simulink model "MHILSimHWImpl"  (R2024a)
settings: Solver=FixedStepDiscrete  StartTime=0.0  StopTime=2e-4  FixedStep=4e-9  RelTol=1e-3
values from neighbouring files (symbols this model uses):
  cfg = tddbl_model    [HILSimModel.m]
undefined symbols (not defined in the file or in its folder): AXI4, dt, hw, ip, Lite, xc7z020clg400
libraries: hdlBasic x1497, hdlUtilities x3, vmcUtilities x1
(part 4 of 11)

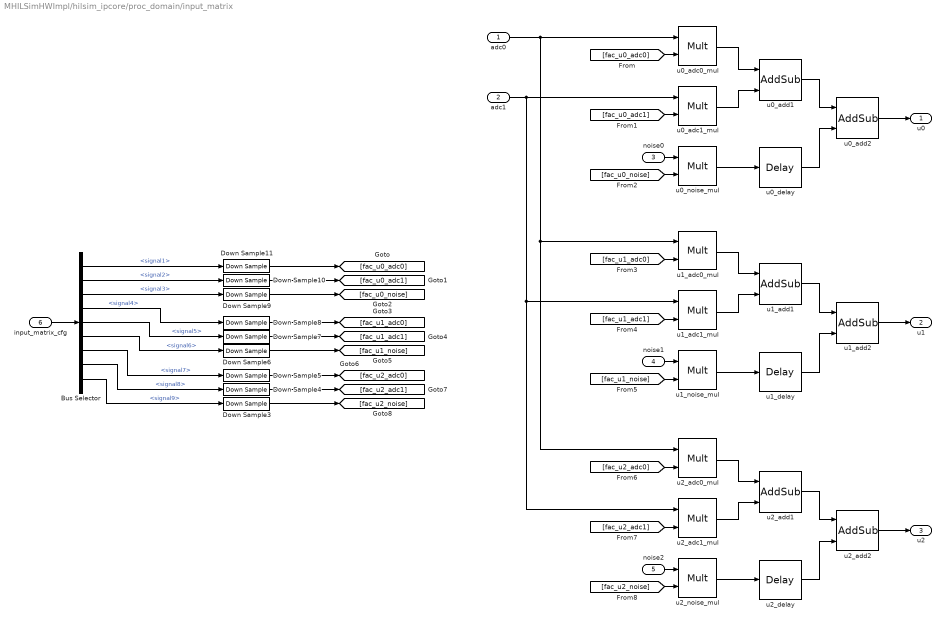
== system MHILSimHWImpl/hilsim_ipcore/proc_domain/input_matrix ==
  adc0 : Inport
  adc1 : Inport  Port=2
  noise0 : Inport  Port=3
  noise1 : Inport  Port=4
  noise2 : Inport  Port=5
  input_matrix_cfg : Inport  Port=6
  Bus Selector : BusSelector  OutputSignals=signal1,signal2,signal3,signal4,signal5,signal6,signal7,signal8,signal9
  Down Sample{3..11} (9 alike) : hdlBasic/Down Sample  sample_ratio=hw.oversample  sample_phase="Last Value of Frame  (most efficient)"  en=off  rst=off  latency=1  XmcBlockStatus=1  maskContainerNames=group1  block_type=dsamp  block_config=sysgen:Downsample_config
  u0_adc0_mul : hdlBasic/Mult  precision=User Defined  arith_type="Signed  (2's comp)"  n_bits=dt.slice.sz  bin_pt=dt.slice.bin  quantization=Truncate  overflow=Wrap  en=off  latency=3  opt_float=off  fp_mult_usage=No Usage  use_behavioral_HDL=off  opt=Speed  use_embedded=on  optimum_pipeline=off  pipeline=on  use_rpm=on  placement_style=Triangular  XmcBlockStatus=1  maskContainerNames=group1  block_type=mult  block_config=sysgen:Mult_config  block_width=598  block_height=876
  u0_adc1_mul : hdlBasic/Mult  precision=User Defined  arith_type="Signed  (2's comp)"  n_bits=dt.slice.sz  bin_pt=dt.slice.bin  quantization=Truncate  overflow=Wrap  en=off  latency=3  opt_float=off  fp_mult_usage=No Usage  use_behavioral_HDL=off  opt=Speed  use_embedded=on  optimum_pipeline=off  pipeline=on  use_rpm=on  placement_style=Triangular  XmcBlockStatus=1  maskContainerNames=group1  block_type=mult  block_config=sysgen:Mult_config  block_width=598  block_height=876
  u0_add1 : hdlBasic/AddSub  mode=Addition  use_carryin=off  use_carryout=off  en=off  latency=1  precision=User Defined  arith_type="Signed  (2's comp)"  n_bits=dt.slice.sz  bin_pt=dt.slice.bin  quantization=Truncate  overflow=Wrap  use_behavioral_HDL=off  hw_selection=Fabric  pipelined=off  XmcBlockStatus=1  maskContainerNames=tabcontainer1  block_type=addsub  block_config=sysgen:Addsub_config
  u0_add2 : hdlBasic/AddSub  mode=Addition  use_carryin=off  use_carryout=off  en=off  latency=1  precision=User Defined  arith_type="Signed  (2's comp)"  n_bits=dt.slice.sz  bin_pt=dt.slice.bin  quantization=Truncate  overflow=Wrap  use_behavioral_HDL=off  hw_selection=Fabric  pipelined=off  XmcBlockStatus=1  maskContainerNames=tabcontainer1  block_type=addsub  block_config=sysgen:Addsub_config
  u0_delay : hdlBasic/Delay  rst=off  en=off  latency=1  reg_retiming=off  XmcBlockStatus=1  maskContainerNames=group1  block_type=delay  block_config=sysgen:Delay_config
  u0_noise_mul : hdlBasic/Mult  precision=User Defined  arith_type="Signed  (2's comp)"  n_bits=dt.slice.sz  bin_pt=dt.slice.bin  quantization=Truncate  overflow=Wrap  en=off  latency=3  opt_float=off  fp_mult_usage=No Usage  use_behavioral_HDL=off  opt=Speed  use_embedded=on  optimum_pipeline=off  pipeline=on  use_rpm=on  placement_style=Triangular  XmcBlockStatus=1  maskContainerNames=group1  block_type=mult  block_config=sysgen:Mult_config  block_width=598  block_height=876
  u1_adc0_mul : hdlBasic/Mult  precision=User Defined  arith_type="Signed  (2's comp)"  n_bits=dt.slice.sz  bin_pt=dt.slice.bin  quantization=Truncate  overflow=Wrap  en=off  latency=3  opt_float=off  fp_mult_usage=No Usage  use_behavioral_HDL=off  opt=Speed  use_embedded=on  optimum_pipeline=off  pipeline=on  use_rpm=on  placement_style=Triangular  XmcBlockStatus=1  maskContainerNames=group1  block_type=mult  block_config=sysgen:Mult_config  block_width=598  block_height=876
  u1_adc1_mul : hdlBasic/Mult  precision=User Defined  arith_type="Signed  (2's comp)"  n_bits=dt.slice.sz  bin_pt=dt.slice.bin  quantization=Truncate  overflow=Wrap  en=off  latency=3  opt_float=off  fp_mult_usage=No Usage  use_behavioral_HDL=off  opt=Speed  use_embedded=on  optimum_pipeline=off  pipeline=on  use_rpm=on  placement_style=Triangular  XmcBlockStatus=1  maskContainerNames=group1  block_type=mult  block_config=sysgen:Mult_config  block_width=598  block_height=876
  u1_add1 : hdlBasic/AddSub  mode=Addition  use_carryin=off  use_carryout=off  en=off  latency=1  precision=User Defined  arith_type="Signed  (2's comp)"  n_bits=dt.slice.sz  bin_pt=dt.slice.bin  quantization=Truncate  overflow=Wrap  use_behavioral_HDL=off  hw_selection=Fabric  pipelined=off  XmcBlockStatus=1  maskContainerNames=tabcontainer1  block_type=addsub  block_config=sysgen:Addsub_config
  u1_add2 : hdlBasic/AddSub  mode=Addition  use_carryin=off  use_carryout=off  en=off  latency=1  precision=User Defined  arith_type="Signed  (2's comp)"  n_bits=dt.slice.sz  bin_pt=dt.slice.bin  quantization=Truncate  overflow=Wrap  use_behavioral_HDL=off  hw_selection=Fabric  pipelined=off  XmcBlockStatus=1  maskContainerNames=tabcontainer1  block_type=addsub  block_config=sysgen:Addsub_config
  u1_delay : hdlBasic/Delay  rst=off  en=off  latency=1  reg_retiming=off  XmcBlockStatus=1  maskContainerNames=group1  block_type=delay  block_config=sysgen:Delay_config
  u1_noise_mul : hdlBasic/Mult  precision=User Defined  arith_type="Signed  (2's comp)"  n_bits=dt.slice.sz  bin_pt=dt.slice.bin  quantization=Truncate  overflow=Wrap  en=off  latency=3  opt_float=off  fp_mult_usage=No Usage  use_behavioral_HDL=off  opt=Speed  use_embedded=on  optimum_pipeline=off  pipeline=on  use_rpm=on  placement_style=Triangular  XmcBlockStatus=1  maskContainerNames=group1  block_type=mult  block_config=sysgen:Mult_config  block_width=598  block_height=876
  u2_adc0_mul : hdlBasic/Mult  precision=User Defined  arith_type="Signed  (2's comp)"  n_bits=dt.slice.sz  bin_pt=dt.slice.bin  quantization=Truncate  overflow=Wrap  en=off  latency=3  opt_float=off  fp_mult_usage=No Usage  use_behavioral_HDL=off  opt=Speed  use_embedded=on  optimum_pipeline=off  pipeline=on  use_rpm=on  placement_style=Triangular  XmcBlockStatus=1  maskContainerNames=group1  block_type=mult  block_config=sysgen:Mult_config  block_width=598  block_height=876
  u2_adc1_mul : hdlBasic/Mult  precision=User Defined  arith_type="Signed  (2's comp)"  n_bits=dt.slice.sz  bin_pt=dt.slice.bin  quantization=Truncate  overflow=Wrap  en=off  latency=3  opt_float=off  fp_mult_usage=No Usage  use_behavioral_HDL=off  opt=Speed  use_embedded=on  optimum_pipeline=off  pipeline=on  use_rpm=on  placement_style=Triangular  XmcBlockStatus=1  maskContainerNames=group1  block_type=mult  block_config=sysgen:Mult_config  block_width=598  block_height=876
  u2_add1 : hdlBasic/AddSub  mode=Addition  use_carryin=off  use_carryout=off  en=off  latency=1  precision=User Defined  arith_type="Signed  (2's comp)"  n_bits=dt.slice.sz  bin_pt=dt.slice.bin  quantization=Truncate  overflow=Wrap  use_behavioral_HDL=off  hw_selection=Fabric  pipelined=off  XmcBlockStatus=1  maskContainerNames=tabcontainer1  block_type=addsub  block_config=sysgen:Addsub_config
  u2_add2 : hdlBasic/AddSub  mode=Addition  use_carryin=off  use_carryout=off  en=off  latency=1  precision=User Defined  arith_type="Signed  (2's comp)"  n_bits=dt.slice.sz  bin_pt=dt.slice.bin  quantization=Truncate  overflow=Wrap  use_behavioral_HDL=off  hw_selection=Fabric  pipelined=off  XmcBlockStatus=1  maskContainerNames=tabcontainer1  block_type=addsub  block_config=sysgen:Addsub_config
  u2_delay : hdlBasic/Delay  rst=off  en=off  latency=1  reg_retiming=off  XmcBlockStatus=1  maskContainerNames=group1  block_type=delay  block_config=sysgen:Delay_config
  u2_noise_mul : hdlBasic/Mult  precision=User Defined  arith_type="Signed  (2's comp)"  n_bits=dt.slice.sz  bin_pt=dt.slice.bin  quantization=Truncate  overflow=Wrap  en=off  latency=3  opt_float=off  fp_mult_usage=No Usage  use_behavioral_HDL=off  opt=Speed  use_embedded=on  optimum_pipeline=off  pipeline=on  use_rpm=on  placement_style=Triangular  XmcBlockStatus=1  maskContainerNames=group1  block_type=mult  block_config=sysgen:Mult_config  block_width=598  block_height=876
  u0 : Outport
  u1 : Outport  Port=2
  u2 : Outport  Port=3
  wires:
  u0_add1/1 -> u0_add2/1
  u0_adc0_mul/1 -> u0_add1/1
  u0_adc1_mul/1 -> u0_add1/2
  u0_noise_mul/1 -> u0_delay/1
  u0_add2/1 -> u0/1
  u1_add1/1 -> u1_add2/1
  u1_adc1_mul/1 -> u1_add1/2
  u1_adc0_mul/1 -> u1_add1/1
  u1_noise_mul/1 -> u1_delay/1
  u2_add1/1 -> u2_add2/1
  u2_adc1_mul/1 -> u2_add1/2
  u2_adc0_mul/1 -> u2_add1/1
  u2_noise_mul/1 -> u2_delay/1
  adc0/1 -> u0_adc0_mul/1, u2_adc0_mul/1, u1_adc0_mul/1
  adc1/1 -> u0_adc1_mul/1, u2_adc1_mul/1, u1_adc1_mul/1
  u1_add2/1 -> u1/1
  u2_add2/1 -> u2/1
  [fac_u0_adc0] -> u0_adc0_mul/2
  [fac_u0_adc1] -> u0_adc1_mul/2
  [fac_u0_noise] -> u0_noise_mul/2
  [fac_u1_adc0] -> u1_adc0_mul/2
  [fac_u1_adc1] -> u1_adc1_mul/2
  [fac_u1_noise] -> u1_noise_mul/2
  [fac_u2_adc0] -> u2_adc0_mul/2
  [fac_u2_noise] -> u2_noise_mul/2
  [fac_u2_adc1] -> u2_adc1_mul/2
  Bus Selector/1 -> Down Sample11/1  "<signal1>"
  Bus Selector/2 -> Down Sample10/1  "<signal2>"
  Bus Selector/3 -> Down Sample9/1  "<signal3>"
  Bus Selector/9 -> Down Sample3/1  "<signal9>"
  Bus Selector/8 -> Down Sample4/1  "<signal8>"
  Bus Selector/7 -> Down Sample5/1  "<signal7>"
  Bus Selector/6 -> Down Sample6/1  "<signal6>"
  Bus Selector/5 -> Down Sample7/1  "<signal5>"
  Bus Selector/4 -> Down Sample8/1  "<signal4>"
  input_matrix_cfg/1 -> Bus Selector/1
  Down Sample3/1 -> [fac_u2_noise]
  Down Sample4/1 -> [fac_u2_adc1]
  Down Sample5/1 -> [fac_u2_adc0]
  Down Sample7/1 -> [fac_u1_adc1]
  Down Sample8/1 -> [fac_u1_adc0]
  Down Sample6/1 -> [fac_u1_noise]
  Down Sample11/1 -> [fac_u0_adc0]
  Down Sample9/1 -> [fac_u0_noise]
  Down Sample10/1 -> [fac_u0_adc1]
  u0_delay/1 -> u0_add2/2
  u1_delay/1 -> u1_add2/2
  u2_delay/1 -> u2_add2/2
  noise0/1 -> u0_noise_mul/1
  noise1/1 -> u1_noise_mul/1
  noise2/1 -> u2_noise_mul/1

== system MHILSimHWImpl/hilsim_ipcore/proc_domain/input_shutoff ==
  enable : Inport
  u0_in : Inport  Port=2
  u1_in : Inport  Port=3
  u2_in : Inport  Port=4
  Constant1 : hdlBasic/Constant  const=0  gui_display_data_type=Fixed-point  arith_type=Signed (2's comp)  n_bits=dt.slice.sz  bin_pt=dt.slice.bin  preci_type=Single  exp_width=8  frac_width=24  explicit_period=off  period=1  XmcBlockStatus=1  maskContainerNames=tabcontainer1  block_type=constant  block_config=sysgen:Constant_config
  Constant2 : hdlBasic/Constant  const=0  gui_display_data_type=Fixed-point  arith_type=Signed (2's comp)  n_bits=dt.slice.sz  bin_pt=dt.slice.bin  preci_type=Single  exp_width=8  frac_width=24  explicit_period=off  period=1  XmcBlockStatus=1  maskContainerNames=tabcontainer1  block_type=constant  block_config=sysgen:Constant_config
  Constant3 : hdlBasic/Constant  const=0  gui_display_data_type=Fixed-point  arith_type=Signed (2's comp)  n_bits=dt.slice.sz  bin_pt=dt.slice.bin  preci_type=Single  exp_width=8  frac_width=24  explicit_period=off  period=1  XmcBlockStatus=1  maskContainerNames=tabcontainer1  block_type=constant  block_config=sysgen:Constant_config
  mux_u0 : hdlBasic/Mux  inputs=2  en=off  latency=0  precision=Full  arith_type=Unsigned  n_bits=16  bin_pt=14  quantization=Truncate  overflow=Wrap  XmcBlockStatus=1  maskContainerNames=tabcontainer1  block_type=mux  block_config=sysgen:Mux_config
  mux_u1 : hdlBasic/Mux  inputs=2  en=off  latency=0  precision=Full  arith_type=Unsigned  n_bits=16  bin_pt=14  quantization=Truncate  overflow=Wrap  XmcBlockStatus=1  maskContainerNames=tabcontainer1  block_type=mux  block_config=sysgen:Mux_config
  mux_u2 : hdlBasic/Mux  inputs=2  en=off  latency=0  precision=Full  arith_type=Unsigned  n_bits=16  bin_pt=14  quantization=Truncate  overflow=Wrap  XmcBlockStatus=1  maskContainerNames=tabcontainer1  block_type=mux  block_config=sysgen:Mux_config
  u0_out : Outport
  u1_out : Outport  Port=2
  u2_out : Outport  Port=3
  wires:
  Constant1/1 -> mux_u0/2
  Constant2/1 -> mux_u1/2
  Constant3/1 -> mux_u2/2
  u0_in/1 -> mux_u0/3
  enable/1 -> mux_u2/1, mux_u1/1, mux_u0/1
  u1_in/1 -> mux_u1/3
  u2_in/1 -> mux_u2/3
  mux_u0/1 -> u0_out/1
  mux_u1/1 -> u1_out/1
  mux_u2/1 -> u2_out/1

== system MHILSimHWImpl/hilsim_ipcore/proc_domain/nlf_lut_configurator ==
  note: Rising-Edge Trigger for Write-Enable
  procclk_lutcfg_addr : Inport
  procclk_lutcfg_data_in : Inport  Port=2
  procclk_lutcfg_we : Inport  Port=3
  cfg_nlf_start : Inport  Port=4
  Constant : hdlBasic/Constant  const=1.0  gui_display_data_type=Boolean  arith_type=Boolean  n_bits=16  bin_pt=14  preci_type=Single  exp_width=8  frac_width=24  explicit_period=off  period=1  XmcBlockStatus=1  maskContainerNames=tabcontainer1  block_type=constant  block_config=sysgen:Constant_config
  Constant1 : hdlBasic/Constant  const=1.0  gui_display_data_type=Fixed-point  arith_type=Unsigned  n_bits=ip.f_nlf.lut_addr_bits  bin_pt=0  preci_type=Single  exp_width=8  frac_width=24  explicit_period=off  period=1  XmcBlockStatus=1  maskContainerNames=tabcontainer1  block_type=constant  block_config=sysgen:Constant_config
  Constant2 : hdlBasic/Constant  const=ip.f_nlf.lut_sz-1  gui_display_data_type=Fixed-point  arith_type=Unsigned  n_bits=ip.f_nlf.lut_addr_bits  bin_pt=0  preci_type=Single  exp_width=8  frac_width=24  explicit_period=off  period=1  XmcBlockStatus=1  maskContainerNames=tabcontainer1  block_type=constant  block_config=sysgen:Constant_config
  Constant3 : hdlBasic/Constant  const=1.0  gui_display_data_type=Boolean  arith_type=Boolean  n_bits=16  bin_pt=14  preci_type=Single  exp_width=8  frac_width=24  explicit_period=off  period=1  XmcBlockStatus=1  maskContainerNames=tabcontainer1  block_type=constant  block_config=sysgen:Constant_config
  Delay : hdlBasic/Delay  rst=off  en=off  latency=1  reg_retiming=off  XmcBlockStatus=1  maskContainerNames=group1  block_type=delay  block_config=sysgen:Delay_config
  Delay1 : hdlBasic/Delay  rst=off  en=off  latency=1  reg_retiming=off  XmcBlockStatus=1  maskContainerNames=group1  block_type=delay  block_config=sysgen:Delay_config
  Mux : hdlBasic/Mux  inputs=2  en=off  latency=0  precision=Full  arith_type=Unsigned  n_bits=16  bin_pt=14  quantization=Truncate  overflow=Wrap  XmcBlockStatus=1  maskContainerNames=tabcontainer1  block_type=mux  block_config=sysgen:Mux_config
  Mux1 : hdlBasic/Mux  inputs=2  en=off  latency=0  precision=Full  arith_type=Unsigned  n_bits=16  bin_pt=14  quantization=Truncate  overflow=Wrap  XmcBlockStatus=1  maskContainerNames=tabcontainer1  block_type=mux  block_config=sysgen:Mux_config
  Register : hdlBasic/Register  init=0  rst=on  en=off  XmcBlockStatus=1  maskContainerNames=tabcontainer1  block_type=register  block_config=sysgen:Register_config
  Register1 : hdlBasic/Register  init=0  rst=on  en=off  XmcBlockStatus=1  maskContainerNames=tabcontainer1  block_type=register  block_config=sysgen:Register_config
  Relational : hdlBasic/Relational  mode=a=b  op_type=Bool  en=off  latency=1  XmcBlockStatus=1  maskContainerNames=tabcontainer1  block_type=relational  block_config=sysgen:Relational_config
  Terminator : Terminator
  addr_counter : hdlBasic/Accumulator  operation=Add  n_bits=ip.f_nlf.lut_addr_bits  overflow=Wrap  scale=1  rst=on  hasbypass=off  en=on  latency=1  msb_inp=100  msb=100  lsb=-100  use_behavioral_HDL=on  implementation=Fabric  XmcBlockStatus=1  maskContainerNames=group3  block_type=accum  block_config=sysgen:Accum_config  block_width=566  block_height=845
  bool_zero : hdlBasic/Constant  const=0  gui_display_data_type=Boolean  arith_type=Boolean  n_bits=16  bin_pt=14  preci_type=Single  exp_width=8  frac_width=24  explicit_period=off  period=1  XmcBlockStatus=1  maskContainerNames=tabcontainer1  block_type=constant  block_config=sysgen:Constant_config
  cfg_we_and : hdlBasic/Logical  logical_function=AND  inputs=2  en=off  latency=0  precision=Full  arith_type=Unsigned  n_bits=16  bin_pt=0  align_bp=on  overflow=[]  quantization=[]  XmcBlockStatus=1  maskContainerNames=tabcontainer1  block_type=logical  block_config=sysgen:Logical_config
  cfg_we_inv : hdlBasic/Inverter  en=off  latency=1  XmcBlockStatus=1  maskContainerNames=group2  block_type=inv  block_config=sysgen:Inverter_config
  tmp_lut : hdlBasic/Dual Port RAM  depth=ip.f_nlf.lut_sz  initVector=cfg.slice1.x_nlf.lut  distributed_mem=Block RAM  init_a=0  init_b=0  rst_a=off  rst_b=off  en_a=off  en_b=off  latency=1  write_mode_A=Read After Write  write_mode_B=Read After Write  explicit_period=[]  period=[]  simulation_type=fast_sim  XmcBlockStatus=1  maskContainerNames=tabcontainer1  block_type=dpram  block_config=sysgen:Dpram_config  optimize=Area
      settings: infoedit=[]
  zero_nlf_din : hdlBasic/Constant  const=0  gui_display_data_type=Fixed-point  arith_type=Signed (2's comp)  n_bits=dt.nlf.sz  bin_pt=dt.nlf.bin  preci_type=Single  exp_width=8  frac_width=24  explicit_period=off  period=1  XmcBlockStatus=1  maskContainerNames=tabcontainer1  block_type=constant  block_config=sysgen:Constant_config
  procclk_cfgbus_addr : Outport
  procclk_cfgbus_data : Outport  Port=2
  procclk_cfgbus_we : Outport  Port=3
  cfg_nlf_done : Outport  Port=4
  wires:
  procclk_lutcfg_data_in/1 -> tmp_lut/2
  procclk_lutcfg_addr/1 -> tmp_lut/1
  tmp_lut/1 -> Terminator/1
  tmp_lut/2 -> procclk_cfgbus_data/1
  cfg_nlf_start/1 -> Register1/2, Mux/1
  Mux/1 -> Register/1
  Register/1 -> addr_counter/3, Delay1/1, Mux/2
  Constant/1 -> Mux/3
  Constant1/1 -> addr_counter/1
  addr_counter/1 -> Delay/1, tmp_lut/4, Relational/1
  Relational/1 -> addr_counter/2, Mux1/1, Register/2  "cfg_nlf_last_addr"
  Constant2/1 -> Relational/2
  bool_zero/1 -> tmp_lut/6
  zero_nlf_din/1 -> tmp_lut/5
  cfg_we_and/1 -> tmp_lut/3
  cfg_we_inv/1 -> cfg_we_and/1
  procclk_lutcfg_we/1 -> cfg_we_and/2, cfg_we_inv/1
  Mux1/1 -> Register1/1
  Register1/1 -> cfg_nlf_done/1, Mux1/2
  Constant3/1 -> Mux1/3
  Delay/1 -> procclk_cfgbus_addr/1
  Delay1/1 -> procclk_cfgbus_we/1

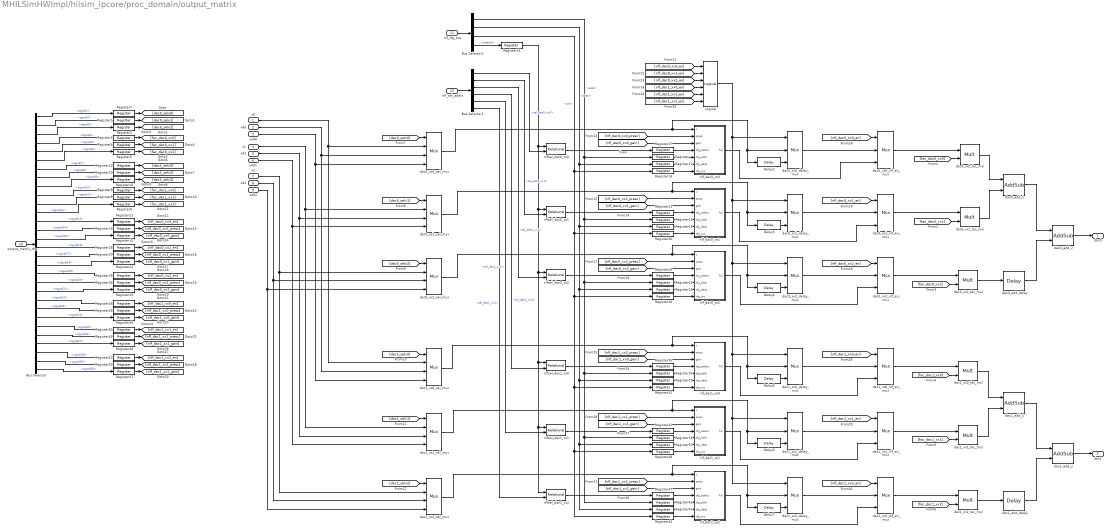
== system MHILSimHWImpl/hilsim_ipcore/proc_domain/output_matrix ==
  x0 : Inport
  xd0 : Inport  Port=2
  xdd0 : Inport  Port=3
  x1 : Inport  Port=4
  xd1 : Inport  Port=5
  xdd1 : Inport  Port=6
  x2 : Inport  Port=7
  xd2 : Inport  Port=8
  xdd2 : Inport  Port=9
  output_matrix_cfg : Inport  Port=10
  nlf_cfg_bus : Inport  Port=11
  nlf_sel_addrs : Inport  Port=12
  Bus Selector : BusSelector  OutputSignals=signal1,signal2,signal3,signal4,signal5,signal6,signal7,signal8,signal9,signal10,signal11,signal12,signal13,signal14,signal15,signal16,signal17,signal18,signal19,signal20,signal21,signal22,signal23,signal24,signal25,signal26,signal27,signal28,signal29,signal30
  Bus Selector1 : BusSelector  OutputSignals=sel_dac0_xx0,sel_dac0_xx1,sel_dac0_xx2,sel_dac1_xx0,sel_dac1_xx1,sel_dac1_xx2
  Bus Selector2 : BusSelector  OutputSignals=addr,data,we,seladdr
  Delay{2..7} (6 alike) : hdlBasic/Delay  rst=off  en=off  latency=12  reg_retiming=off  XmcBlockStatus=1  maskContainerNames=group1  block_type=delay  block_config=sysgen:Delay_config
  Logical : hdlBasic/Logical  logical_function=OR  inputs=6  en=off  latency=0  precision=Full  arith_type=Unsigned  n_bits=16  bin_pt=0  align_bp=on  overflow=[]  quantization=[]  XmcBlockStatus=1  maskContainerNames=tabcontainer1  block_type=logical  block_config=sysgen:Logical_config
  Register{,1..54} (55 alike) : hdlBasic/Register  init=0  rst=off  en=off  XmcBlockStatus=1  maskContainerNames=tabcontainer1  block_type=register  block_config=sysgen:Register_config
  dac0_add_1 : hdlBasic/AddSub  mode=Addition  use_carryin=off  use_carryout=off  en=off  latency=1  precision=User Defined  arith_type="Signed  (2's comp)"  n_bits=dt.slice.sz  bin_pt=dt.slice.bin  quantization=Truncate  overflow=Wrap  use_behavioral_HDL=off  hw_selection=Fabric  pipelined=off  XmcBlockStatus=1  maskContainerNames=tabcontainer1  block_type=addsub  block_config=sysgen:Addsub_config
  dac0_add_2 : hdlBasic/AddSub  mode=Addition  use_carryin=off  use_carryout=off  en=off  latency=1  precision=User Defined  arith_type="Signed  (2's comp)"  n_bits=dt.slice.sz  bin_pt=dt.slice.bin  quantization=Truncate  overflow=Wrap  use_behavioral_HDL=off  hw_selection=Fabric  pipelined=off  XmcBlockStatus=1  maskContainerNames=tabcontainer1  block_type=addsub  block_config=sysgen:Addsub_config
  dac0_add_delay : hdlBasic/Delay  rst=off  en=off  latency=1  reg_retiming=off  XmcBlockStatus=1  maskContainerNames=group1  block_type=delay  block_config=sysgen:Delay_config
  dac0_xx0_delay_mux : hdlBasic/Mux  inputs=2  en=off  latency=0  precision=Full  arith_type=Unsigned  n_bits=16  bin_pt=14  quantization=Truncate  overflow=Wrap  XmcBlockStatus=1  maskContainerNames=tabcontainer1  block_type=mux  block_config=sysgen:Mux_config
  dac0_xx0_fac_mul : hdlBasic/Mult  precision=User Defined  arith_type="Signed  (2's comp)"  n_bits=dt.slice.sz  bin_pt=dt.slice.bin  quantization=Truncate  overflow=Wrap  en=off  latency=3  opt_float=off  fp_mult_usage=No Usage  use_behavioral_HDL=off  opt=Speed  use_embedded=on  optimum_pipeline=off  pipeline=on  use_rpm=on  placement_style=Triangular  XmcBlockStatus=1  maskContainerNames=group1  block_type=mult  block_config=sysgen:Mult_config  block_width=598  block_height=876
  dac0_xx0_nlf_en_mux : hdlBasic/Mux  inputs=2  en=off  latency=1  precision=Full  arith_type=Unsigned  n_bits=16  bin_pt=14  quantization=Truncate  overflow=Wrap  XmcBlockStatus=1  maskContainerNames=tabcontainer1  block_type=mux  block_config=sysgen:Mux_config
  dac0_xx0_sel_mux : hdlBasic/Mux  inputs=3  en=off  latency=1  precision=Full  arith_type=Unsigned  n_bits=16  bin_pt=14  quantization=Truncate  overflow=Wrap  XmcBlockStatus=1  maskContainerNames=tabcontainer1  block_type=mux  block_config=sysgen:Mux_config
  dac0_xx1_delay_mux : hdlBasic/Mux  inputs=2  en=off  latency=0  precision=Full  arith_type=Unsigned  n_bits=16  bin_pt=14  quantization=Truncate  overflow=Wrap  XmcBlockStatus=1  maskContainerNames=tabcontainer1  block_type=mux  block_config=sysgen:Mux_config
  dac0_xx1_fac_mul : hdlBasic/Mult  precision=User Defined  arith_type="Signed  (2's comp)"  n_bits=dt.slice.sz  bin_pt=dt.slice.bin  quantization=Truncate  overflow=Wrap  en=off  latency=3  opt_float=off  fp_mult_usage=No Usage  use_behavioral_HDL=off  opt=Speed  use_embedded=on  optimum_pipeline=off  pipeline=on  use_rpm=on  placement_style=Triangular  XmcBlockStatus=1  maskContainerNames=group1  block_type=mult  block_config=sysgen:Mult_config  block_width=598  block_height=876
  dac0_xx1_nlf_en_mux : hdlBasic/Mux  inputs=2  en=off  latency=1  precision=Full  arith_type=Unsigned  n_bits=16  bin_pt=14  quantization=Truncate  overflow=Wrap  XmcBlockStatus=1  maskContainerNames=tabcontainer1  block_type=mux  block_config=sysgen:Mux_config
  dac0_xx1_sel_mux : hdlBasic/Mux  inputs=3  en=off  latency=1  precision=Full  arith_type=Unsigned  n_bits=16  bin_pt=14  quantization=Truncate  overflow=Wrap  XmcBlockStatus=1  maskContainerNames=tabcontainer1  block_type=mux  block_config=sysgen:Mux_config
  dac0_xx2_delay_mux : hdlBasic/Mux  inputs=2  en=off  latency=0  precision=Full  arith_type=Unsigned  n_bits=16  bin_pt=14  quantization=Truncate  overflow=Wrap  XmcBlockStatus=1  maskContainerNames=tabcontainer1  block_type=mux  block_config=sysgen:Mux_config
  dac0_xx2_fac_mul : hdlBasic/Mult  precision=User Defined  arith_type="Signed  (2's comp)"  n_bits=dt.slice.sz  bin_pt=dt.slice.bin  quantization=Truncate  overflow=Wrap  en=off  latency=3  opt_float=off  fp_mult_usage=No Usage  use_behavioral_HDL=off  opt=Speed  use_embedded=on  optimum_pipeline=off  pipeline=on  use_rpm=on  placement_style=Triangular  XmcBlockStatus=1  maskContainerNames=group1  block_type=mult  block_config=sysgen:Mult_config  block_width=598  block_height=876
  dac0_xx2_nlf_en_mux : hdlBasic/Mux  inputs=2  en=off  latency=1  precision=Full  arith_type=Unsigned  n_bits=16  bin_pt=14  quantization=Truncate  overflow=Wrap  XmcBlockStatus=1  maskContainerNames=tabcontainer1  block_type=mux  block_config=sysgen:Mux_config
  dac0_xx2_sel_mux : hdlBasic/Mux  inputs=3  en=off  latency=1  precision=Full  arith_type=Unsigned  n_bits=16  bin_pt=14  quantization=Truncate  overflow=Wrap  XmcBlockStatus=1  maskContainerNames=tabcontainer1  block_type=mux  block_config=sysgen:Mux_config
  dac1_add_1 : hdlBasic/AddSub  mode=Addition  use_carryin=off  use_carryout=off  en=off  latency=1  precision=User Defined  arith_type="Signed  (2's comp)"  n_bits=dt.slice.sz  bin_pt=dt.slice.bin  quantization=Truncate  overflow=Wrap  use_behavioral_HDL=off  hw_selection=Fabric  pipelined=off  XmcBlockStatus=1  maskContainerNames=tabcontainer1  block_type=addsub  block_config=sysgen:Addsub_config
  dac1_add_2 : hdlBasic/AddSub  mode=Addition  use_carryin=off  use_carryout=off  en=off  latency=1  precision=User Defined  arith_type="Signed  (2's comp)"  n_bits=dt.slice.sz  bin_pt=dt.slice.bin  quantization=Truncate  overflow=Wrap  use_behavioral_HDL=off  hw_selection=Fabric  pipelined=off  XmcBlockStatus=1  maskContainerNames=tabcontainer1  block_type=addsub  block_config=sysgen:Addsub_config
  dac1_add_delay : hdlBasic/Delay  rst=off  en=off  latency=1  reg_retiming=off  XmcBlockStatus=1  maskContainerNames=group1  block_type=delay  block_config=sysgen:Delay_config
  dac1_xx0_delay_mux : hdlBasic/Mux  inputs=2  en=off  latency=0  precision=Full  arith_type=Unsigned  n_bits=16  bin_pt=14  quantization=Truncate  overflow=Wrap  XmcBlockStatus=1  maskContainerNames=tabcontainer1  block_type=mux  block_config=sysgen:Mux_config
  dac1_xx0_fac_mul : hdlBasic/Mult  precision=User Defined  arith_type="Signed  (2's comp)"  n_bits=dt.slice.sz  bin_pt=dt.slice.bin  quantization=Truncate  overflow=Wrap  en=off  latency=3  opt_float=off  fp_mult_usage=No Usage  use_behavioral_HDL=off  opt=Speed  use_embedded=on  optimum_pipeline=off  pipeline=on  use_rpm=on  placement_style=Triangular  XmcBlockStatus=1  maskContainerNames=group1  block_type=mult  block_config=sysgen:Mult_config  block_width=598  block_height=876
  dac1_xx0_nlf_en_mux : hdlBasic/Mux  inputs=2  en=off  latency=1  precision=Full  arith_type=Unsigned  n_bits=16  bin_pt=14  quantization=Truncate  overflow=Wrap  XmcBlockStatus=1  maskContainerNames=tabcontainer1  block_type=mux  block_config=sysgen:Mux_config
  dac1_xx0_sel_mux : hdlBasic/Mux  inputs=3  en=off  latency=1  precision=Full  arith_type=Unsigned  n_bits=16  bin_pt=14  quantization=Truncate  overflow=Wrap  XmcBlockStatus=1  maskContainerNames=tabcontainer1  block_type=mux  block_config=sysgen:Mux_config
  dac1_xx1_delay_mux : hdlBasic/Mux  inputs=2  en=off  latency=0  precision=Full  arith_type=Unsigned  n_bits=16  bin_pt=14  quantization=Truncate  overflow=Wrap  XmcBlockStatus=1  maskContainerNames=tabcontainer1  block_type=mux  block_config=sysgen:Mux_config
  dac1_xx1_fac_mul : hdlBasic/Mult  precision=User Defined  arith_type="Signed  (2's comp)"  n_bits=dt.slice.sz  bin_pt=dt.slice.bin  quantization=Truncate  overflow=Wrap  en=off  latency=3  opt_float=off  fp_mult_usage=No Usage  use_behavioral_HDL=off  opt=Speed  use_embedded=on  optimum_pipeline=off  pipeline=on  use_rpm=on  placement_style=Triangular  XmcBlockStatus=1  maskContainerNames=group1  block_type=mult  block_config=sysgen:Mult_config  block_width=598  block_height=876
  dac1_xx1_nlf_en_mux : hdlBasic/Mux  inputs=2  en=off  latency=1  precision=Full  arith_type=Unsigned  n_bits=16  bin_pt=14  quantization=Truncate  overflow=Wrap  XmcBlockStatus=1  maskContainerNames=tabcontainer1  block_type=mux  block_config=sysgen:Mux_config
  dac1_xx1_sel_mux : hdlBasic/Mux  inputs=3  en=off  latency=1  precision=Full  arith_type=Unsigned  n_bits=16  bin_pt=14  quantization=Truncate  overflow=Wrap  XmcBlockStatus=1  maskContainerNames=tabcontainer1  block_type=mux  block_config=sysgen:Mux_config
  dac1_xx2_delay_mux : hdlBasic/Mux  inputs=2  en=off  latency=0  precision=Full  arith_type=Unsigned  n_bits=16  bin_pt=14  quantization=Truncate  overflow=Wrap  XmcBlockStatus=1  maskContainerNames=tabcontainer1  block_type=mux  block_config=sysgen:Mux_config
  dac1_xx2_fac_mul : hdlBasic/Mult  precision=User Defined  arith_type="Signed  (2's comp)"  n_bits=dt.slice.sz  bin_pt=dt.slice.bin  quantization=Truncate  overflow=Wrap  en=off  latency=3  opt_float=off  fp_mult_usage=No Usage  use_behavioral_HDL=off  opt=Speed  use_embedded=on  optimum_pipeline=off  pipeline=on  use_rpm=on  placement_style=Triangular  XmcBlockStatus=1  maskContainerNames=group1  block_type=mult  block_config=sysgen:Mult_config  block_width=598  block_height=876
  dac1_xx2_nlf_en_mux : hdlBasic/Mux  inputs=2  en=off  latency=1  precision=Full  arith_type=Unsigned  n_bits=16  bin_pt=14  quantization=Truncate  overflow=Wrap  XmcBlockStatus=1  maskContainerNames=tabcontainer1  block_type=mux  block_config=sysgen:Mux_config
  dac1_xx2_sel_mux : hdlBasic/Mux  inputs=3  en=off  latency=1  precision=Full  arith_type=Unsigned  n_bits=16  bin_pt=14  quantization=Truncate  overflow=Wrap  XmcBlockStatus=1  maskContainerNames=tabcontainer1  block_type=mux  block_config=sysgen:Mux_config
  nlf_dac0_xx0 : Subsystem
  nlf_dac0_xx1 : Subsystem
  nlf_dac0_xx2 : Subsystem
  nlf_dac1_xx0 : Subsystem
  nlf_dac1_xx1 : Subsystem
  nlf_dac1_xx2 : Subsystem
  nlfsel_dac0_xx0 : hdlBasic/Relational  mode=a=b  op_type=Bool  en=off  latency=1  XmcBlockStatus=1  maskContainerNames=tabcontainer1  block_type=relational  block_config=sysgen:Relational_config
  nlfsel_dac0_xx1 : hdlBasic/Relational  mode=a=b  op_type=Bool  en=off  latency=1  XmcBlockStatus=1  maskContainerNames=tabcontainer1  block_type=relational  block_config=sysgen:Relational_config
  nlfsel_dac0_xx2 : hdlBasic/Relational  mode=a=b  op_type=Bool  en=off  latency=1  XmcBlockStatus=1  maskContainerNames=tabcontainer1  block_type=relational  block_config=sysgen:Relational_config
  nlfsel_dac1_xx0 : hdlBasic/Relational  mode=a=b  op_type=Bool  en=off  latency=1  XmcBlockStatus=1  maskContainerNames=tabcontainer1  block_type=relational  block_config=sysgen:Relational_config
  nlfsel_dac1_xx1 : hdlBasic/Relational  mode=a=b  op_type=Bool  en=off  latency=1  XmcBlockStatus=1  maskContainerNames=tabcontainer1  block_type=relational  block_config=sysgen:Relational_config
  nlfsel_dac1_xx2 : hdlBasic/Relational  mode=a=b  op_type=Bool  en=off  latency=1  XmcBlockStatus=1  maskContainerNames=tabcontainer1  block_type=relational  block_config=sysgen:Relational_config
  dac0 : Outport
  dac1 : Outport  Port=2
  wires:
  dac0_xx0_sel_mux/1 -> nlf_dac0_xx0/1(x), Delay2/1, dac0_xx0_delay_mux/2
  [fac_dac0_xx0] -> dac0_xx0_fac_mul/2
  [fac_dac0_xx1] -> dac0_xx1_fac_mul/2
  [fac_dac0_xx2] -> dac0_xx2_fac_mul/2
  dac0_xx0_fac_mul/1 -> dac0_add_1/1
  dac0_xx1_fac_mul/1 -> dac0_add_1/2
  dac0_add_1/1 -> dac0_add_2/1
  dac0_xx2_fac_mul/1 -> dac0_add_delay/1
  dac0_add_2/1 -> dac0/1
  dac1_add_1/1 -> dac1_add_2/1
  dac1_xx0_fac_mul/1 -> dac1_add_1/1
  dac1_xx1_fac_mul/1 -> dac1_add_1/2
  [fac_dac1_xx1] -> dac1_xx1_fac_mul/2
  [fac_dac1_xx0] -> dac1_xx0_fac_mul/2
  [fac_dac1_xx2] -> dac1_xx2_fac_mul/2
  dac1_add_2/1 -> dac1/1
  dac1_xx2_fac_mul/1 -> dac1_add_delay/1
  [dac0_selx0] -> dac0_xx0_sel_mux/1
  [dac0_selx1] -> dac0_xx1_sel_mux/1
  [dac0_selx2] -> dac0_xx2_sel_mux/1
  [dac1_selx0] -> dac1_xx0_sel_mux/1
  [dac1_selx1] -> dac1_xx1_sel_mux/1
  [dac1_selx2] -> dac1_xx2_sel_mux/1
  x0/1 -> dac1_xx0_sel_mux/2, dac0_xx0_sel_mux/2
  xd0/1 -> dac1_xx0_sel_mux/3, dac0_xx0_sel_mux/3
  x1/1 -> dac1_xx1_sel_mux/2, dac0_xx1_sel_mux/2
  xd1/1 -> dac1_xx1_sel_mux/3, dac0_xx1_sel_mux/3
  x2/1 -> dac1_xx2_sel_mux/2, dac0_xx2_sel_mux/2
  xd2/1 -> dac1_xx2_sel_mux/3, dac0_xx2_sel_mux/3
  Bus Selector/1 -> Register7/1  "<signal1>"
  Bus Selector/2 -> Register1/1  "<signal2>"
  Bus Selector/12 -> Register6/1  "<signal12>"
  Bus Selector/11 -> Register8/1  "<signal11>"
  Bus Selector/10 -> Register9/1  "<signal10>"
  Bus Selector/9 -> Register10/1  "<signal9>"
  Bus Selector/8 -> Register11/1  "<signal8>"
  Bus Selector/7 -> Register12/1  "<signal7>"
  Bus Selector/6 -> Register5/1  "<signal6>"
  Bus Selector/5 -> Register4/1  "<signal5>"
  Bus Selector/4 -> Register3/1  "<signal4>"
  Bus Selector/3 -> Register2/1  "<signal3>"
  output_matrix_cfg/1 -> Bus Selector/1
  dac0_add_delay/1 -> dac0_add_2/2
  dac1_add_delay/1 -> dac1_add_2/2
  Register7/1 -> [dac0_selx0]
  Register1/1 -> [dac0_selx1]
  Register2/1 -> [dac0_selx2]
  Register3/1 -> [fac_dac0_xx0]
  Register4/1 -> [fac_dac0_xx1]
  Register5/1 -> [fac_dac0_xx2]
  Register6/1 -> [fac_dac1_xx2]
  Register8/1 -> [fac_dac1_xx1]
  Register9/1 -> [fac_dac1_xx0]
  Register10/1 -> [dac1_selx2]
  Register11/1 -> [dac1_selx1]
  Register12/1 -> [dac1_selx0]
  Register/1 -> nlf_dac0_xx0/5(cfg_addr)
  [nlf_dac0_xx0_gain] -> nlf_dac0_xx0/3(gain)
  Register14/1 -> nlf_dac0_xx0/7(cfg_we)
  Register13/1 -> nlf_dac0_xx0/6(cfg_data)
  [nlf_dac0_xx0_presc] -> nlf_dac0_xx0/2(presc)
  Register17/1 -> nlf_dac0_xx0/4(cfg_select)
  dac0_xx0_delay_mux/1 -> dac0_xx0_nlf_en_mux/2
  Delay2/1 -> dac0_xx0_delay_mux/3
  nlf_dac0_xx0/1(f(x)) -> dac0_xx0_nlf_en_mux/3
  nlfsel_dac0_xx0/1 -> Register17/1
  Register20/1 -> nlf_dac0_xx1/7(cfg_we)
  Register23/1 -> nlf_dac0_xx1/4(cfg_select)
  [nlf_dac0_xx1_gain] -> nlf_dac0_xx1/3(gain)
  dac0_xx1_delay_mux/1 -> dac0_xx1_nlf_en_mux/2
  Register19/1 -> nlf_dac0_xx1/6(cfg_data)
  [nlf_dac0_xx1_presc] -> nlf_dac0_xx1/2(presc)
  nlf_dac0_xx1/1(f(x)) -> dac0_xx1_nlf_en_mux/3
  Register18/1 -> nlf_dac0_xx1/5(cfg_addr)
  Delay3/1 -> dac0_xx1_delay_mux/3
  dac0_xx1_sel_mux/1 -> nlf_dac0_xx1/1(x), Delay3/1, dac0_xx1_delay_mux/2
  nlf_dac0_xx2/1(f(x)) -> dac0_xx2_nlf_en_mux/3
  Register25/1 -> nlf_dac0_xx2/6(cfg_data)
  dac0_xx2_delay_mux/1 -> dac0_xx2_nlf_en_mux/2
  [nlf_dac0_xx2_gain] -> nlf_dac0_xx2/3(gain)
  Register29/1 -> nlf_dac0_xx2/4(cfg_select)
  Register26/1 -> nlf_dac0_xx2/7(cfg_we)
  [nlf_dac0_xx2_presc] -> nlf_dac0_xx2/2(presc)
  Register24/1 -> nlf_dac0_xx2/5(cfg_addr)
  Delay4/1 -> dac0_xx2_delay_mux/3
  dac0_xx2_sel_mux/1 -> nlf_dac0_xx2/1(x), Delay4/1, dac0_xx2_delay_mux/2
  dac0_xx0_nlf_en_mux/1 -> dac0_xx0_fac_mul/1
  dac0_xx1_nlf_en_mux/1 -> dac0_xx1_fac_mul/1
  dac0_xx2_nlf_en_mux/1 -> dac0_xx2_fac_mul/1
  [nlf_dac0_xx0_en] -> dac0_xx0_nlf_en_mux/1
  [nlf_dac0_xx1_en] -> dac0_xx1_nlf_en_mux/1
  [nlf_dac0_xx2_en] -> dac0_xx2_nlf_en_mux/1
  [nlf_dac0_xx0_en] -> Logical/1
  [nlf_dac0_xx1_en] -> Logical/2
  [nlf_dac0_xx2_en] -> Logical/3
  Register32/1 -> nlf_dac1_xx0/7(cfg_we)
  Register35/1 -> nlf_dac1_xx0/4(cfg_select)
  [nlf_dac1_xx0_gain] -> nlf_dac1_xx0/3(gain)
  dac1_xx0_sel_mux/1 -> nlf_dac1_xx0/1(x), Delay5/1, dac1_xx0_delay_mux/2
  dac1_xx0_delay_mux/1 -> dac1_xx0_nlf_en_mux/2
  Register30/1 -> nlf_dac1_xx0/5(cfg_addr)
  Register31/1 -> nlf_dac1_xx0/6(cfg_data)
  nlf_dac1_xx0/1(f(x)) -> dac1_xx0_nlf_en_mux/3
  [nlf_dac1_xx0_presc] -> nlf_dac1_xx0/2(presc)
  [nlf_dac1_xx0_en] -> dac1_xx0_nlf_en_mux/1
  Delay5/1 -> dac1_xx0_delay_mux/3
  dac1_xx0_nlf_en_mux/1 -> dac1_xx0_fac_mul/1
  Register38/1 -> nlf_dac1_xx1/7(cfg_we)
  Register41/1 -> nlf_dac1_xx1/4(cfg_select)
  [nlf_dac1_xx1_gain] -> nlf_dac1_xx1/3(gain)
  dac1_xx1_sel_mux/1 -> nlf_dac1_xx1/1(x), Delay6/1, dac1_xx1_delay_mux/2
  dac1_xx1_delay_mux/1 -> dac1_xx1_nlf_en_mux/2
  Register36/1 -> nlf_dac1_xx1/5(cfg_addr)
  Register37/1 -> nlf_dac1_xx1/6(cfg_data)
  nlf_dac1_xx1/1(f(x)) -> dac1_xx1_nlf_en_mux/3
  [nlf_dac1_xx1_presc] -> nlf_dac1_xx1/2(presc)
  [nlf_dac1_xx1_en] -> dac1_xx1_nlf_en_mux/1
  Delay6/1 -> dac1_xx1_delay_mux/3
  dac1_xx1_nlf_en_mux/1 -> dac1_xx1_fac_mul/1
  Register44/1 -> nlf_dac1_xx2/7(cfg_we)
  Register47/1 -> nlf_dac1_xx2/4(cfg_select)
  [nlf_dac1_xx2_gain] -> nlf_dac1_xx2/3(gain)
  dac1_xx2_sel_mux/1 -> nlf_dac1_xx2/1(x), Delay7/1, dac1_xx2_delay_mux/2
  dac1_xx2_delay_mux/1 -> dac1_xx2_nlf_en_mux/2
  Register42/1 -> nlf_dac1_xx2/5(cfg_addr)
  Register43/1 -> nlf_dac1_xx2/6(cfg_data)
  nlf_dac1_xx2/1(f(x)) -> dac1_xx2_nlf_en_mux/3
  [nlf_dac1_xx2_presc] -> nlf_dac1_xx2/2(presc)
  [nlf_dac1_xx2_en] -> dac1_xx2_nlf_en_mux/1
  Bus Selector2/2 -> Register13/1, Register43/1, Register37/1, Register31/1, Register25/1, Register19/1  "<data>"
  Delay7/1 -> dac1_xx2_delay_mux/3
  dac1_xx2_nlf_en_mux/1 -> dac1_xx2_fac_mul/1
  Bus Selector2/1 -> Register42/1, Register36/1, Register30/1, Register24/1, Register18/1, Register/1  "<addr>"
  Logical/1 -> dac1_xx2_delay_mux/1, dac1_xx1_delay_mux/1, dac1_xx0_delay_mux/1, dac0_xx2_delay_mux/1, dac0_xx1_delay_mux/1, dac0_xx0_delay_mux/1
  Bus Selector2/3 -> Register14/1, Register44/1, Register38/1, Register32/1, Register26/1, Register20/1  "<we>"
  [nlf_dac1_xx1_en] -> Logical/5
  [nlf_dac1_xx2_en] -> Logical/6
  [nlf_dac1_xx0_en] -> Logical/4
  Register21/1 -> [nlf_dac0_xx0_en]
  Register16/1 -> [nlf_dac0_xx0_presc]
  Register15/1 -> [nlf_dac0_xx0_gain]
  Register28/1 -> [nlf_dac0_xx1_en]
  Register27/1 -> [nlf_dac0_xx1_presc]
  Register22/1 -> [nlf_dac0_xx1_gain]
  Register39/1 -> [nlf_dac0_xx2_en]
  Register33/1 -> [nlf_dac0_xx2_gain]
  Register34/1 -> [nlf_dac0_xx2_presc]
  Register50/1 -> [nlf_dac1_xx1_en]
  Register53/1 -> [nlf_dac1_xx2_en]
  Register45/1 -> [nlf_dac1_xx0_presc]
  Register52/1 -> [nlf_dac1_xx2_presc]
  Register40/1 -> [nlf_dac1_xx0_gain]
  Register48/1 -> [nlf_dac1_xx1_gain]
  Register51/1 -> [nlf_dac1_xx2_gain]
  Register49/1 -> [nlf_dac1_xx1_presc]
  Register46/1 -> [nlf_dac1_xx0_en]
  Bus Selector/13 -> Register21/1  "<signal13>"
  Bus Selector/14 -> Register16/1  "<signal14>"
  Bus Selector/15 -> Register15/1  "<signal15>"
  Bus Selector/16 -> Register28/1  "<signal16>"
  Bus Selector/17 -> Register27/1  "<signal17>"
  Bus Selector/18 -> Register22/1  "<signal18>"
  Bus Selector/19 -> Register39/1  "<signal19>"
  Bus Selector/20 -> Register34/1  "<signal20>"
  Bus Selector/21 -> Register33/1  "<signal21>"
  Bus Selector/22 -> Register46/1  "<signal22>"
  Bus Selector/23 -> Register45/1  "<signal23>"
  Bus Selector/24 -> Register40/1  "<signal24>"
  Bus Selector/25 -> Register50/1  "<signal25>"
  Bus Selector/26 -> Register49/1  "<signal26>"
  Bus Selector/27 -> Register48/1  "<signal27>"
  Bus Selector/28 -> Register53/1  "<signal28>"
  Bus Selector/29 -> Register52/1  "<signal29>"
  Bus Selector/30 -> Register51/1  "<signal30>"
  xdd0/1 -> dac1_xx0_sel_mux/4, dac0_xx0_sel_mux/4
  xdd1/1 -> dac1_xx1_sel_mux/4, dac0_xx1_sel_mux/4
  xdd2/1 -> dac1_xx2_sel_mux/4, dac0_xx2_sel_mux/4
  nlf_sel_addrs/1 -> Bus Selector1/1
  Bus Selector1/1 -> nlfsel_dac0_xx0/2  "<sel_dac0_xx0>"
  nlfsel_dac0_xx1/1 -> Register23/1
  Bus Selector1/2 -> nlfsel_dac0_xx1/2  "<sel_dac0_xx1>"
  nlfsel_dac0_xx2/1 -> Register29/1
  Bus Selector1/3 -> nlfsel_dac0_xx2/2  "<sel_dac0_xx2>"
  nlf_cfg_bus/1 -> Bus Selector2/1
  Bus Selector2/4 -> Register54/1  "<seladdr>"
  Register54/1 -> nlfsel_dac1_xx2/1, nlfsel_dac1_xx1/1, nlfsel_dac1_xx0/1, nlfsel_dac0_xx2/1, nlfsel_dac0_xx1/1, nlfsel_dac0_xx0/1
  nlfsel_dac1_xx0/1 -> Register35/1
  Bus Selector1/4 -> nlfsel_dac1_xx0/2  "<sel_dac1_xx0>"
  nlfsel_dac1_xx1/1 -> Register41/1
  nlfsel_dac1_xx2/1 -> Register47/1
  Bus Selector1/5 -> nlfsel_dac1_xx1/2  "<sel_dac1_xx1>"
  Bus Selector1/6 -> nlfsel_dac1_xx2/2  "<sel_dac1_xx2>"

== system MHILSimHWImpl/hilsim_ipcore/proc_domain/output_switch ==
  enable : Inport
  dac0_in : Inport  Port=2
  dac1_in : Inport  Port=3
  Constant1 : hdlBasic/Constant  const=0  gui_display_data_type=Fixed-point  arith_type=Signed (2's comp)  n_bits=dt.slice.sz  bin_pt=dt.slice.bin  preci_type=Single  exp_width=8  frac_width=24  explicit_period=off  period=1  XmcBlockStatus=1  maskContainerNames=tabcontainer1  block_type=constant  block_config=sysgen:Constant_config
  Constant3 : hdlBasic/Constant  const=0  gui_display_data_type=Fixed-point  arith_type=Signed (2's comp)  n_bits=dt.slice.sz  bin_pt=dt.slice.bin  preci_type=Single  exp_width=8  frac_width=24  explicit_period=off  period=1  XmcBlockStatus=1  maskContainerNames=tabcontainer1  block_type=constant  block_config=sysgen:Constant_config
  Mux1 : hdlBasic/Mux  inputs=2  en=off  latency=0  precision=Full  arith_type=Unsigned  n_bits=16  bin_pt=14  quantization=Truncate  overflow=Wrap  XmcBlockStatus=1  maskContainerNames=tabcontainer1  block_type=mux  block_config=sysgen:Mux_config
  Mux2 : hdlBasic/Mux  inputs=2  en=off  latency=0  precision=Full  arith_type=Unsigned  n_bits=16  bin_pt=14  quantization=Truncate  overflow=Wrap  XmcBlockStatus=1  maskContainerNames=tabcontainer1  block_type=mux  block_config=sysgen:Mux_config
  dac0_out : Outport
  dac1_out : Outport  Port=2
  wires:
  Constant3/1 -> Mux1/2
  Constant1/1 -> Mux2/2
  dac0_in/1 -> Mux1/3
  dac1_in/1 -> Mux2/3
  Mux1/1 -> dac0_out/1
  Mux2/1 -> dac1_out/1
  enable/1 -> Mux2/1, Mux1/1

== system MHILSimHWImpl/hilsim_ipcore/proc_domain/sel_addrs_adc ==
  Bus Creator : BusCreator  Inputs=2
  Constant : hdlBasic/Constant  const=ip.nlfaddr.adc0  gui_display_data_type=Fixed-point  arith_type=Unsigned  n_bits=8  bin_pt=0  preci_type=Single  exp_width=8  frac_width=24  explicit_period=off  period=1  XmcBlockStatus=1  maskContainerNames=tabcontainer1  block_type=constant  block_config=sysgen:Constant_config
  Constant1 : hdlBasic/Constant  const=ip.nlfaddr.adc1  gui_display_data_type=Fixed-point  arith_type=Unsigned  n_bits=8  bin_pt=0  preci_type=Single  exp_width=8  frac_width=24  explicit_period=off  period=1  XmcBlockStatus=1  maskContainerNames=tabcontainer1  block_type=constant  block_config=sysgen:Constant_config
  nlf_sel_addrs : Outport
  wires:
  Bus Creator/1 -> nlf_sel_addrs/1
  Constant/1 -> Bus Creator/1  "sel_adc0"
  Constant1/1 -> Bus Creator/2  "sel_adc1"

== system MHILSimHWImpl/hilsim_ipcore/proc_domain/sel_addrs_output_matrix ==
  Bus Creator : BusCreator  Inputs=6
  Constant : hdlBasic/Constant  const=ip.nlfaddr.dac0_xx0  gui_display_data_type=Fixed-point  arith_type=Unsigned  n_bits=8  bin_pt=0  preci_type=Single  exp_width=8  frac_width=24  explicit_period=off  period=1  XmcBlockStatus=1  maskContainerNames=tabcontainer1  block_type=constant  block_config=sysgen:Constant_config
  Constant1 : hdlBasic/Constant  const=ip.nlfaddr.dac0_xx1  gui_display_data_type=Fixed-point  arith_type=Unsigned  n_bits=8  bin_pt=0  preci_type=Single  exp_width=8  frac_width=24  explicit_period=off  period=1  XmcBlockStatus=1  maskContainerNames=tabcontainer1  block_type=constant  block_config=sysgen:Constant_config
  Constant2 : hdlBasic/Constant  const=ip.nlfaddr.dac0_xx2  gui_display_data_type=Fixed-point  arith_type=Unsigned  n_bits=8  bin_pt=0  preci_type=Single  exp_width=8  frac_width=24  explicit_period=off  period=1  XmcBlockStatus=1  maskContainerNames=tabcontainer1  block_type=constant  block_config=sysgen:Constant_config
  Constant3 : hdlBasic/Constant  const=ip.nlfaddr.dac1_xx0  gui_display_data_type=Fixed-point  arith_type=Unsigned  n_bits=8  bin_pt=0  preci_type=Single  exp_width=8  frac_width=24  explicit_period=off  period=1  XmcBlockStatus=1  maskContainerNames=tabcontainer1  block_type=constant  block_config=sysgen:Constant_config
  Constant4 : hdlBasic/Constant  const=ip.nlfaddr.dac1_xx1  gui_display_data_type=Fixed-point  arith_type=Unsigned  n_bits=8  bin_pt=0  preci_type=Single  exp_width=8  frac_width=24  explicit_period=off  period=1  XmcBlockStatus=1  maskContainerNames=tabcontainer1  block_type=constant  block_config=sysgen:Constant_config
  Constant5 : hdlBasic/Constant  const=ip.nlfaddr.dac1_xx2  gui_display_data_type=Fixed-point  arith_type=Unsigned  n_bits=8  bin_pt=0  preci_type=Single  exp_width=8  frac_width=24  explicit_period=off  period=1  XmcBlockStatus=1  maskContainerNames=tabcontainer1  block_type=constant  block_config=sysgen:Constant_config
  nlf_sel_addrs : Outport
  wires:
  Bus Creator/1 -> nlf_sel_addrs/1
  Constant/1 -> Bus Creator/1  "sel_dac0_xx0"
  Constant1/1 -> Bus Creator/2  "sel_dac0_xx1"
  Constant2/1 -> Bus Creator/3  "sel_dac0_xx2"
  Constant3/1 -> Bus Creator/4  "sel_dac1_xx0"
  Constant4/1 -> Bus Creator/5  "sel_dac1_xx1"
  Constant5/1 -> Bus Creator/6  "sel_dac1_xx2"

== system MHILSimHWImpl/hilsim_ipcore/proc_domain/sel_addrs_slice_0 ==
  Bus Creator : BusCreator  Inputs=6
  Constant : hdlBasic/Constant  const=ip.nlfaddr.slice0_u0  gui_display_data_type=Fixed-point  arith_type=Unsigned  n_bits=8  bin_pt=0  preci_type=Single  exp_width=8  frac_width=24  explicit_period=off  period=1  XmcBlockStatus=1  maskContainerNames=tabcontainer1  block_type=constant  block_config=sysgen:Constant_config
  Constant1 : hdlBasic/Constant  const=ip.nlfaddr.slice0_u1  gui_display_data_type=Fixed-point  arith_type=Unsigned  n_bits=8  bin_pt=0  preci_type=Single  exp_width=8  frac_width=24  explicit_period=off  period=1  XmcBlockStatus=1  maskContainerNames=tabcontainer1  block_type=constant  block_config=sysgen:Constant_config
  Constant2 : hdlBasic/Constant  const=ip.nlfaddr.slice0_x0  gui_display_data_type=Fixed-point  arith_type=Unsigned  n_bits=8  bin_pt=0  preci_type=Single  exp_width=8  frac_width=24  explicit_period=off  period=1  XmcBlockStatus=1  maskContainerNames=tabcontainer1  block_type=constant  block_config=sysgen:Constant_config
  Constant3 : hdlBasic/Constant  const=ip.nlfaddr.slice0_x1  gui_display_data_type=Fixed-point  arith_type=Unsigned  n_bits=8  bin_pt=0  preci_type=Single  exp_width=8  frac_width=24  explicit_period=off  period=1  XmcBlockStatus=1  maskContainerNames=tabcontainer1  block_type=constant  block_config=sysgen:Constant_config
  Constant4 : hdlBasic/Constant  const=ip.nlfaddr.slice0_xd0  gui_display_data_type=Fixed-point  arith_type=Unsigned  n_bits=8  bin_pt=0  preci_type=Single  exp_width=8  frac_width=24  explicit_period=off  period=1  XmcBlockStatus=1  maskContainerNames=tabcontainer1  block_type=constant  block_config=sysgen:Constant_config
  Constant5 : hdlBasic/Constant  const=ip.nlfaddr.slice0_xd1  gui_display_data_type=Fixed-point  arith_type=Unsigned  n_bits=8  bin_pt=0  preci_type=Single  exp_width=8  frac_width=24  explicit_period=off  period=1  XmcBlockStatus=1  maskContainerNames=tabcontainer1  block_type=constant  block_config=sysgen:Constant_config
  nlf_sel_addrs : Outport
  wires:
  Bus Creator/1 -> nlf_sel_addrs/1
  Constant/1 -> Bus Creator/1  "sel_u0"
  Constant1/1 -> Bus Creator/2  "sel_u1"
  Constant2/1 -> Bus Creator/3  "sel_x0"
  Constant3/1 -> Bus Creator/4  "sel_x1"
  Constant4/1 -> Bus Creator/5  "sel_xd0"
  Constant5/1 -> Bus Creator/6  "sel_xd1"

== system MHILSimHWImpl/hilsim_ipcore/proc_domain/sel_addrs_slice_1 ==
  Bus Creator : BusCreator  Inputs=6
  Constant : hdlBasic/Constant  const=ip.nlfaddr.slice1_u0  gui_display_data_type=Fixed-point  arith_type=Unsigned  n_bits=8  bin_pt=0  preci_type=Single  exp_width=8  frac_width=24  explicit_period=off  period=1  XmcBlockStatus=1  maskContainerNames=tabcontainer1  block_type=constant  block_config=sysgen:Constant_config
  Constant1 : hdlBasic/Constant  const=ip.nlfaddr.slice1_u1  gui_display_data_type=Fixed-point  arith_type=Unsigned  n_bits=8  bin_pt=0  preci_type=Single  exp_width=8  frac_width=24  explicit_period=off  period=1  XmcBlockStatus=1  maskContainerNames=tabcontainer1  block_type=constant  block_config=sysgen:Constant_config
  Constant2 : hdlBasic/Constant  const=ip.nlfaddr.slice1_x0  gui_display_data_type=Fixed-point  arith_type=Unsigned  n_bits=8  bin_pt=0  preci_type=Single  exp_width=8  frac_width=24  explicit_period=off  period=1  XmcBlockStatus=1  maskContainerNames=tabcontainer1  block_type=constant  block_config=sysgen:Constant_config
  Constant3 : hdlBasic/Constant  const=ip.nlfaddr.slice1_x1  gui_display_data_type=Fixed-point  arith_type=Unsigned  n_bits=8  bin_pt=0  preci_type=Single  exp_width=8  frac_width=24  explicit_period=off  period=1  XmcBlockStatus=1  maskContainerNames=tabcontainer1  block_type=constant  block_config=sysgen:Constant_config
  Constant4 : hdlBasic/Constant  const=ip.nlfaddr.slice1_xd0  gui_display_data_type=Fixed-point  arith_type=Unsigned  n_bits=8  bin_pt=0  preci_type=Single  exp_width=8  frac_width=24  explicit_period=off  period=1  XmcBlockStatus=1  maskContainerNames=tabcontainer1  block_type=constant  block_config=sysgen:Constant_config
  Constant5 : hdlBasic/Constant  const=ip.nlfaddr.slice1_xd1  gui_display_data_type=Fixed-point  arith_type=Unsigned  n_bits=8  bin_pt=0  preci_type=Single  exp_width=8  frac_width=24  explicit_period=off  period=1  XmcBlockStatus=1  maskContainerNames=tabcontainer1  block_type=constant  block_config=sysgen:Constant_config
  nlf_sel_addrs : Outport
  wires:
  Bus Creator/1 -> nlf_sel_addrs/1
  Constant/1 -> Bus Creator/1  "sel_u0"
  Constant1/1 -> Bus Creator/2  "sel_u1"
  Constant2/1 -> Bus Creator/3  "sel_x0"
  Constant3/1 -> Bus Creator/4  "sel_x1"
  Constant4/1 -> Bus Creator/5  "sel_xd0"
  Constant5/1 -> Bus Creator/6  "sel_xd1"
